simulink model "case6"  (R2024b)
settings: Solver=FixedStepAuto  StartTime=0  StopTime=1  FixedStep=1e-7  RelTol=1e-3
values from neighbouring files (symbols this model uses):
  SG_D_1_D = 0.01056    [IEEE9_case_parameters.m]    (also in case1_parameters.m; case2_parameters.m; case3_parameters.m; case4_parameters.m)
  SG_D_1_EnableSaturation = 0    [IEEE9_case_parameters.m]    (also in case1_parameters.m; case2_parameters.m; case3_parameters.m; case4_parameters.m)
  SG_D_1_f0 = 60    [IEEE9_case_parameters.m]    (also in case1_parameters.m; case2_parameters.m; case3_parameters.m; case4_parameters.m)
  SG_D_1_H = 7.5    [IEEE9_case_parameters.m]    (also in case1_parameters.m; case2_parameters.m; case3_parameters.m; case4_parameters.m)
  SG_D_1_K_A = 20    [IEEE9_case_parameters.m]    (also in case1_parameters.m; case2_parameters.m; case3_parameters.m; case4_parameters.m)
  SG_D_1_K_E = 1.000000e+1    (= 10)    [IEEE9_case_parameters.m]    (also in case1_parameters.m; case2_parameters.m; case3_parameters.m; case4_parameters.m)
  SG_D_1_K_F = 2.363    [IEEE9_case_parameters.m]    (also in case1_parameters.m; case2_parameters.m; case3_parameters.m; case4_parameters.m)
  SG_D_1_K_s = 0.5    [IEEE9_case_parameters.m]    (also in case1_parameters.m = 5; case2_parameters.m = 5; case3_parameters.m = 5; case4_parameters.m = 5)
  SG_D_1_R_a = 0.001088    [IEEE9_case_parameters.m]    (also in case1_parameters.m; case2_parameters.m; case3_parameters.m; case4_parameters.m)
  SG_D_1_S_A = 1    [IEEE9_case_parameters.m]    (also in case1_parameters.m; case2_parameters.m; case3_parameters.m; case4_parameters.m)
  SG_D_1_S_B = 0.103    [IEEE9_case_parameters.m]    (also in case1_parameters.m; case2_parameters.m; case3_parameters.m; case4_parameters.m)
  SG_D_1_S_N = 10.659857    [IEEE9_case_parameters.m]    (also in case1_parameters.m; case2_parameters.m; case3_parameters.m; case4_parameters.m)
  SG_D_1_SpeedPara = 200    [IEEE9_case_parameters.m]    (also in case1_parameters.m; case2_parameters.m; case3_parameters.m; case4_parameters.m)
  SG_D_1_T_0 = 0.720173    [IEEE9_case_parameters.m]    (also in case1_parameters.m = 0.755522; case2_parameters.m = 0.808931; case3_parameters.m = 0.869402; case4_parameters.m = 0.729316)
  SG_D_1_T_1 = 0.3    [IEEE9_case_parameters.m]    (also in case1_parameters.m; case2_parameters.m; case3_parameters.m; case4_parameters.m)
  SG_D_1_T_2 = 0.05    [IEEE9_case_parameters.m]    (also in case1_parameters.m; case2_parameters.m; case3_parameters.m; case4_parameters.m)
  SG_D_1_T_3 = 0.02    [IEEE9_case_parameters.m]    (also in case1_parameters.m; case2_parameters.m; case3_parameters.m; case4_parameters.m)
  SG_D_1_T_4 = 0.005    [IEEE9_case_parameters.m]    (also in case1_parameters.m; case2_parameters.m; case3_parameters.m; case4_parameters.m)
  SG_D_1_T_A = 0.02    [IEEE9_case_parameters.m]    (also in case1_parameters.m; case2_parameters.m; case3_parameters.m; case4_parameters.m)
  SG_D_1_T_dd = 8.000000e+0    (= 8)    [IEEE9_case_parameters.m]    (also in case1_parameters.m; case2_parameters.m; case3_parameters.m; case4_parameters.m)
  SG_D_1_T_ddd = 0.04    [IEEE9_case_parameters.m]    (also in case1_parameters.m; case2_parameters.m; case3_parameters.m; case4_parameters.m)
  SG_D_1_T_E = 0.314    [IEEE9_case_parameters.m]    (also in case1_parameters.m; case2_parameters.m; case3_parameters.m; case4_parameters.m)
  SG_D_1_T_F = 0.35    [IEEE9_case_parameters.m]    (also in case1_parameters.m; case2_parameters.m; case3_parameters.m; case4_parameters.m)
  SG_D_1_T_qd = 0.8    [IEEE9_case_parameters.m]    (also in case1_parameters.m; case2_parameters.m; case3_parameters.m; case4_parameters.m)
  SG_D_1_T_qdd = 0.02    [IEEE9_case_parameters.m]    (also in case1_parameters.m; case2_parameters.m; case3_parameters.m; case4_parameters.m)
  SG_D_1_T_speed = 0.1    [IEEE9_case_parameters.m]    (also in case1_parameters.m = 200; case2_parameters.m = 200; case3_parameters.m = 200; case4_parameters.m = 200)
  SG_D_1_T_w = 0.5    [IEEE9_case_parameters.m]    (also in case1_parameters.m; case2_parameters.m; case3_parameters.m; case4_parameters.m)
  SG_D_1_V_ref = 1.990276    [IEEE9_case_parameters.m]    (also in case1_parameters.m = 2.042296; case2_parameters.m = 2.051388; case3_parameters.m = 2.089584; case4_parameters.m = 2.01845)
  SG_D_1_w_ref = 376.991118    [IEEE9_case_parameters.m]    (also in case1_parameters.m; case2_parameters.m; case3_parameters.m; case4_parameters.m)
  SG_D_1_wb = 6.000000e+1    (= 60)    [IEEE9_case_parameters.m]    (also in case1_parameters.m; case2_parameters.m; case3_parameters.m; case4_parameters.m)
  SG_D_1_x_d = 1.9    [IEEE9_case_parameters.m]    (also in case1_parameters.m; case2_parameters.m; case3_parameters.m; case4_parameters.m)
  SG_D_1_x_dd = 0.302    [IEEE9_case_parameters.m]    (also in case1_parameters.m; case2_parameters.m; case3_parameters.m; case4_parameters.m)
  SG_D_1_x_ddd = 0.204    [IEEE9_case_parameters.m]    (also in case1_parameters.m; case2_parameters.m; case3_parameters.m; case4_parameters.m)
  SG_D_1_x_l = 0.05    [IEEE9_case_parameters.m]    (also in case1_parameters.m; case2_parameters.m; case3_parameters.m; case4_parameters.m)
  SG_D_1_x_q = 1.3    [IEEE9_case_parameters.m]    (also in case1_parameters.m; case2_parameters.m; case3_parameters.m; case4_parameters.m)
  SG_D_1_x_qd = 0.5    [IEEE9_case_parameters.m]    (also in case1_parameters.m; case2_parameters.m; case3_parameters.m; case4_parameters.m)
  SG_D_1_x_qdd = 0.3    [IEEE9_case_parameters.m]    (also in case1_parameters.m; case2_parameters.m; case3_parameters.m; case4_parameters.m)
  SG_D_2_D = 0.02    [IEEE9_case_parameters.m]    (also in case1_parameters.m; case2_parameters.m; case3_parameters.m; case4_parameters.m)
  SG_D_2_EnableSaturation = 0    [IEEE9_case_parameters.m]    (also in case1_parameters.m; case2_parameters.m; case3_parameters.m; case4_parameters.m)
  SG_D_2_f0 = 60    [IEEE9_case_parameters.m]    (also in case1_parameters.m; case2_parameters.m; case3_parameters.m; case4_parameters.m)
  SG_D_2_H = 8.000000e+0    (= 8)    [IEEE9_case_parameters.m]    (also in case1_parameters.m; case2_parameters.m; case3_parameters.m; case4_parameters.m)
  SG_D_2_K_A = 20    [IEEE9_case_parameters.m]    (also in case1_parameters.m; case2_parameters.m; case3_parameters.m; case4_parameters.m)
  SG_D_2_K_E = 1.000000e+1    (= 10)    [IEEE9_case_parameters.m]    (also in case1_parameters.m; case2_parameters.m; case3_parameters.m; case4_parameters.m)
  SG_D_2_K_F = 2.363    [IEEE9_case_parameters.m]    (also in case1_parameters.m; case2_parameters.m; case3_parameters.m; case4_parameters.m)
  SG_D_2_K_s = 0.5    [IEEE9_case_parameters.m]    (also in case1_parameters.m = 4; case2_parameters.m = 4; case3_parameters.m = 4; case4_parameters.m = 4)
  SG_D_2_R_a = 0.001088    [IEEE9_case_parameters.m]    (also in case1_parameters.m; case2_parameters.m; case3_parameters.m; case4_parameters.m)
  SG_D_2_S_A = 1    [IEEE9_case_parameters.m]    (also in case1_parameters.m; case2_parameters.m; case3_parameters.m; case4_parameters.m)
  SG_D_2_S_B = 0.103    [IEEE9_case_parameters.m]    (also in case1_parameters.m; case2_parameters.m; case3_parameters.m; case4_parameters.m)
  SG_D_2_S_N = 10.659857    [IEEE9_case_parameters.m]    (also in case1_parameters.m; case2_parameters.m; case3_parameters.m; case4_parameters.m)
  SG_D_2_SpeedPara = 200    [IEEE9_case_parameters.m]    (also in case1_parameters.m; case2_parameters.m; case3_parameters.m; case4_parameters.m)
  SG_D_2_T_0 = 1.632913    [IEEE9_case_parameters.m]    (also in case1_parameters.m = 1.632925; case2_parameters.m = 1.632915; case3_parameters.m = 1.632914; case4_parameters.m = 1.632927)
  SG_D_2_T_1 = 0.2    [IEEE9_case_parameters.m]    (also in case1_parameters.m; case2_parameters.m; case3_parameters.m; case4_parameters.m)
  SG_D_2_T_2 = 0.05    [IEEE9_case_parameters.m]    (also in case1_parameters.m; case2_parameters.m; case3_parameters.m; case4_parameters.m)
  SG_D_2_T_3 = 0.02    [IEEE9_case_parameters.m]    (also in case1_parameters.m; case2_parameters.m; case3_parameters.m; case4_parameters.m)
  SG_D_2_T_4 = 0.005    [IEEE9_case_parameters.m]    (also in case1_parameters.m; case2_parameters.m; case3_parameters.m; case4_parameters.m)
  SG_D_2_T_A = 0.02    [IEEE9_case_parameters.m]    (also in case1_parameters.m; case2_parameters.m; case3_parameters.m; case4_parameters.m)
  SG_D_2_T_dd = 7.9    [IEEE9_case_parameters.m]    (also in case1_parameters.m; case2_parameters.m; case3_parameters.m; case4_parameters.m)
  SG_D_2_T_ddd = 0.04    [IEEE9_case_parameters.m]    (also in case1_parameters.m; case2_parameters.m; case3_parameters.m; case4_parameters.m)
  SG_D_2_T_E = 0.314    [IEEE9_case_parameters.m]    (also in case1_parameters.m; case2_parameters.m; case3_parameters.m; case4_parameters.m)
  SG_D_2_T_F = 0.35    [IEEE9_case_parameters.m]    (also in case1_parameters.m; case2_parameters.m; case3_parameters.m; case4_parameters.m)
  SG_D_2_T_qd = 0.8    [IEEE9_case_parameters.m]    (also in case1_parameters.m; case2_parameters.m; case3_parameters.m; case4_parameters.m)
  SG_D_2_T_qdd = 0.015    [IEEE9_case_parameters.m]    (also in case1_parameters.m; case2_parameters.m; case3_parameters.m; case4_parameters.m)
  SG_D_2_T_speed = 0.1    [IEEE9_case_parameters.m]    (also in case1_parameters.m = 150; case2_parameters.m = 150; case3_parameters.m = 150; case4_parameters.m = 150)
  SG_D_2_T_w = 0.35    [IEEE9_case_parameters.m]    (also in case1_parameters.m; case2_parameters.m; case3_parameters.m; case4_parameters.m)
  SG_D_2_V_ref = 2.58547    [IEEE9_case_parameters.m]    (also in case1_parameters.m = 2.597896; case2_parameters.m = 2.587136; case3_parameters.m = 2.586042; case4_parameters.m = 2.599679)
  SG_D_2_w_ref = 376.991118    [IEEE9_case_parameters.m]    (also in case1_parameters.m; case2_parameters.m; case3_parameters.m; case4_parameters.m)
  SG_D_2_wb = 6.000000e+1    (= 60)    [IEEE9_case_parameters.m]    (also in case1_parameters.m; case2_parameters.m; case3_parameters.m; case4_parameters.m)
  SG_D_2_x_d = 1.8    [IEEE9_case_parameters.m]    (also in case1_parameters.m; case2_parameters.m; case3_parameters.m; case4_parameters.m)
  SG_D_2_x_dd = 0.302    [IEEE9_case_parameters.m]    (also in case1_parameters.m; case2_parameters.m; case3_parameters.m; case4_parameters.m)
  SG_D_2_x_ddd = 0.204    [IEEE9_case_parameters.m]    (also in case1_parameters.m; case2_parameters.m; case3_parameters.m; case4_parameters.m)
  SG_D_2_x_l = 0.05    [IEEE9_case_parameters.m]    (also in case1_parameters.m; case2_parameters.m; case3_parameters.m; case4_parameters.m)
  SG_D_2_x_q = 1.25    [IEEE9_case_parameters.m]    (also in case1_parameters.m; case2_parameters.m; case3_parameters.m; case4_parameters.m)
  SG_D_2_x_qd = 0.5    [IEEE9_case_parameters.m]    (also in case1_parameters.m; case2_parameters.m; case3_parameters.m; case4_parameters.m)
  SG_D_2_x_qdd = 0.3    [IEEE9_case_parameters.m]    (also in case1_parameters.m; case2_parameters.m; case3_parameters.m; case4_parameters.m)
  SG_D_3_D = 0.02    [IEEE9_case_parameters.m]    (also in case1_parameters.m; case2_parameters.m; case3_parameters.m; case4_parameters.m)
  SG_D_3_EnableSaturation = 0    [IEEE9_case_parameters.m]    (also in case1_parameters.m; case2_parameters.m; case3_parameters.m; case4_parameters.m)
  SG_D_3_f0 = 60    [IEEE9_case_parameters.m]    (also in case1_parameters.m; case2_parameters.m; case3_parameters.m; case4_parameters.m)
  SG_D_3_H = 7.7    [IEEE9_case_parameters.m]    (also in case1_parameters.m; case2_parameters.m; case3_parameters.m; case4_parameters.m)
  SG_D_3_K_A = 20    [IEEE9_case_parameters.m]    (also in case1_parameters.m; case2_parameters.m; case3_parameters.m; case4_parameters.m)
  SG_D_3_K_E = 1.000000e+1    (= 10)    [IEEE9_case_parameters.m]    (also in case1_parameters.m; case2_parameters.m; case3_parameters.m; case4_parameters.m)
  SG_D_3_K_F = 2.363    [IEEE9_case_parameters.m]    (also in case1_parameters.m; case2_parameters.m; case3_parameters.m; case4_parameters.m)
  SG_D_3_K_s = 0.2    [IEEE9_case_parameters.m]    (also in case1_parameters.m = 2; case2_parameters.m = 2; case3_parameters.m = 2; case4_parameters.m = 2)
  SG_D_3_R_a = 0.001088    [IEEE9_case_parameters.m]    (also in case1_parameters.m; case2_parameters.m; case3_parameters.m; case4_parameters.m)
  SG_D_3_S_A = 1    [IEEE9_case_parameters.m]    (also in case1_parameters.m; case2_parameters.m; case3_parameters.m; case4_parameters.m)
  SG_D_3_S_B = 0.103    [IEEE9_case_parameters.m]    (also in case1_parameters.m; case2_parameters.m; case3_parameters.m; case4_parameters.m)
  SG_D_3_S_N = 10.659857    [IEEE9_case_parameters.m]    (also in case1_parameters.m; case2_parameters.m; case3_parameters.m; case4_parameters.m)
  SG_D_3_SpeedPara = 200    [IEEE9_case_parameters.m]    (also in case1_parameters.m; case2_parameters.m; case3_parameters.m; case4_parameters.m)
  SG_D_3_T_0 = 0.850788    [IEEE9_case_parameters.m]    (also in case1_parameters.m = 0.850786; case2_parameters.m = 0.850787; case3_parameters.m; case4_parameters.m = 0.850786)
  SG_D_3_T_1 = 0.2    [IEEE9_case_parameters.m]    (also in case1_parameters.m; case2_parameters.m; case3_parameters.m; case4_parameters.m)
  SG_D_3_T_2 = 0.05    [IEEE9_case_parameters.m]    (also in case1_parameters.m; case2_parameters.m; case3_parameters.m; case4_parameters.m)
  SG_D_3_T_3 = 0.02    [IEEE9_case_parameters.m]    (also in case1_parameters.m; case2_parameters.m; case3_parameters.m; case4_parameters.m)
  SG_D_3_T_4 = 0.005    [IEEE9_case_parameters.m]    (also in case1_parameters.m; case2_parameters.m; case3_parameters.m; case4_parameters.m)
  SG_D_3_T_A = 0.02    [IEEE9_case_parameters.m]    (also in case1_parameters.m; case2_parameters.m; case3_parameters.m; case4_parameters.m)
  SG_D_3_T_dd = 8.1    [IEEE9_case_parameters.m]    (also in case1_parameters.m; case2_parameters.m; case3_parameters.m; case4_parameters.m)
  SG_D_3_T_ddd = 0.04    [IEEE9_case_parameters.m]    (also in case1_parameters.m; case2_parameters.m; case3_parameters.m; case4_parameters.m)
  SG_D_3_T_E = 0.314    [IEEE9_case_parameters.m]    (also in case1_parameters.m; case2_parameters.m; case3_parameters.m; case4_parameters.m)
  SG_D_3_T_F = 0.35    [IEEE9_case_parameters.m]    (also in case1_parameters.m; case2_parameters.m; case3_parameters.m; case4_parameters.m)
  SG_D_3_T_qd = 0.8    [IEEE9_case_parameters.m]    (also in case1_parameters.m; case2_parameters.m; case3_parameters.m; case4_parameters.m)
  SG_D_3_T_qdd = 0.015    [IEEE9_case_parameters.m]    (also in case1_parameters.m; case2_parameters.m; case3_parameters.m; case4_parameters.m)
  SG_D_3_T_speed = 0.1    [IEEE9_case_parameters.m]    (also in case1_parameters.m = 180; case2_parameters.m = 180; case3_parameters.m = 180; case4_parameters.m = 180)
  SG_D_3_T_w = 0.4    [IEEE9_case_parameters.m]    (also in case1_parameters.m; case2_parameters.m; case3_parameters.m; case4_parameters.m)
  SG_D_3_V_ref = 1.892727    [IEEE9_case_parameters.m]    (also in case1_parameters.m = 1.906439; case2_parameters.m = 1.895535; case3_parameters.m = 1.892105; case4_parameters.m = 1.906598)
  SG_D_3_w_ref = 376.991118    [IEEE9_case_parameters.m]    (also in case1_parameters.m; case2_parameters.m; case3_parameters.m; case4_parameters.m)
  SG_D_3_wb = 6.000000e+1    (= 60)    [IEEE9_case_parameters.m]    (also in case1_parameters.m; case2_parameters.m; case3_parameters.m; case4_parameters.m)
  SG_D_3_x_d = 1.85    [IEEE9_case_parameters.m]    (also in case1_parameters.m; case2_parameters.m; case3_parameters.m; case4_parameters.m)
  SG_D_3_x_dd = 0.302    [IEEE9_case_parameters.m]    (also in case1_parameters.m; case2_parameters.m; case3_parameters.m; case4_parameters.m)
  SG_D_3_x_ddd = 0.204    [IEEE9_case_parameters.m]    (also in case1_parameters.m; case2_parameters.m; case3_parameters.m; case4_parameters.m)
  SG_D_3_x_l = 0.05    [IEEE9_case_parameters.m]    (also in case1_parameters.m; case2_parameters.m; case3_parameters.m; case4_parameters.m)
  SG_D_3_x_q = 1.2    [IEEE9_case_parameters.m]    (also in case1_parameters.m; case2_parameters.m; case3_parameters.m; case4_parameters.m)
  SG_D_3_x_qd = 0.5    [IEEE9_case_parameters.m]    (also in case1_parameters.m; case2_parameters.m; case3_parameters.m; case4_parameters.m)
  SG_D_3_x_qdd = 0.3    [IEEE9_case_parameters.m]    (also in case1_parameters.m; case2_parameters.m; case3_parameters.m; case4_parameters.m)
(part 7 of 12)

== system case6/SG_D_2/T_e_SG_D_2_block ==
  note: T_e_SG_D_2 in case6
      | $-\frac{\psi _{d,\mathrm{SG},D,2}\,\left(\psi _{q,\mathrm{SG},D,2}+\frac{\psi _{\mathrm{gq},\mathrm{SG},D,2}\,\left(x_{l}-x_{\mathrm{qdd}}\right)}{x_{l}-x_{\mathrm{qd}}}+\frac{\psi _{\mathrm{kq},\mathrm{SG},D,2}\,\left(x_{\mathrm{qd}}-x_{\mathrm{qdd}}\right)}{x_{l}-x_{\mathrm{qd}}}\right)}{x_{\mathrm{qdd}}}-\frac{\psi _{q,\mathrm{SG},D,2}\,\left(\frac{\psi _{\mathrm{1d},\mathrm{SG},D,2}\,\left(x_{\mathrm{dd}}-x_{\mathrm{ddd}}\right)}{x_{\mathrm{dd}}-x_{l}}-\psi _{d,\mathrm{SG},D,2}+\frac{\psi _{\mathrm{fd},\mathrm{SG},D,2}\,\left(x_{\mathrm{ddd}}-x_{l}\right)}{x_{\mathrm{dd}}-x_{l}}\right)}{x_{\mathrm{ddd}}}$
      | Automatically generated on 2025-10-31 19:18:38 .
  State_psi_d_SG_D_2_01b1a : Inport
  State_psi_gq_SG_D_2_1bd12 : Inport  Port=2
  State_psi_kq_SG_D_2_bf31f : Inport  Port=3
  State_psi_q_SG_D_2_aa98c : Inport  Port=4
  State_psi_q_SG_D_2_0c973 : Inport  Port=5
  State_psi_1d_SG_D_2_e8fde : Inport  Port=6
  State_psi_d_SG_D_2_d0b7a : Inport  Port=7
  State_psi_fd_SG_D_2_ce60b : Inport  Port=8
  Add_2ea7c : Sum
  Add_58bf2 : Sum
  Add_62b30 : Sum
  Add_77a84 : Sum
  Add_e7f98 : Sum
  Add_ea79d : Sum
  Constant_-1_06b6f : Constant  Value=-1
  Constant_-1_114dd : Constant  Value=-1
  Constant_-1_7138b : Constant  Value=-1
  Constant_-1_a1c06 : Constant  Value=-1
  Constant_-1_a700d : Constant  Value=-1
  Constant_x_dd_42f1d : Constant  Value=x_dd
  Constant_x_dd_d85ca : Constant  Value=x_dd
  Constant_x_dd_e0bf0 : Constant  Value=x_dd
  Constant_x_ddd_1e571 : Constant  Value=x_ddd
  Constant_x_ddd_ded06 : Constant  Value=x_ddd
  Constant_x_ddd_ec3b1 : Constant  Value=x_ddd
  Constant_x_l_240e4 : Constant  Value=x_l
  Constant_x_l_3c621 : Constant  Value=x_l
  Constant_x_l_3dcae : Constant  Value=x_l
  Constant_x_l_641a0 : Constant  Value=x_l
  Constant_x_l_8f250 : Constant  Value=x_l
  Constant_x_l_c203d : Constant  Value=x_l
  Constant_x_qd_7d39f : Constant  Value=x_qd
  Constant_x_qd_7eab2 : Constant  Value=x_qd
  Constant_x_qd_8d281 : Constant  Value=x_qd
  Constant_x_qdd_04778 : Constant  Value=x_qdd
  Constant_x_qdd_c9475 : Constant  Value=x_qdd
  Constant_x_qdd_cbb36 : Constant  Value=x_qdd
  Divide_0e157 : Product  Inputs=*/
  Divide_439bb : Product  Inputs=*/
  Divide_8fe5f : Product  Inputs=*/
  Divide_9cb31 : Product  Inputs=*/
  Divide_bf510 : Product  Inputs=*/
  Divide_dccf5 : Product  Inputs=*/
  Product_0b598 : Product
  Product_45b7f : Product
  Product_57456 : Product
  Product_7b54c : Product
  Product_85705 : Product
  Product_8a2e1 : Product
  Product_978bc : Product
  Product_abe4b : Product
  Product_bbeb9 : Product
  Product_c2988 : Product
  Product_d39eb : Product
  Subtract_09de7 : Sum  Inputs=+-
  Subtract_192ee : Sum  Inputs=+-
  Subtract_23775 : Sum  Inputs=+-
  Subtract_362ee : Sum  Inputs=+-
  Subtract_5663d : Sum  Inputs=+-
  Subtract_7336a : Sum  Inputs=+-
  Subtract_ea491 : Sum  Inputs=+-
  Blockout_T_e_SG_D_2_2a19a : Outport
  wires:
  Constant_-1_7138b/1 -> Product_abe4b/1
  Divide_9cb31/1 -> Subtract_09de7/1
  Constant_-1_114dd/1 -> Product_d39eb/1
  Constant_x_l_8f250/1 -> Product_d39eb/2
  Constant_x_qd_7d39f/1 -> Subtract_362ee/1
  Product_57456/1 -> Divide_9cb31/1
  Product_d39eb/1 -> Add_58bf2/1
  Divide_8fe5f/1 -> Subtract_ea491/2
  Constant_x_qdd_c9475/1 -> Subtract_362ee/2
  Constant_x_qdd_cbb36/1 -> Divide_bf510/2
  Constant_x_ddd_ded06/1 -> Subtract_192ee/2
  Constant_x_qdd_04778/1 -> Add_58bf2/2
  Constant_x_l_240e4/1 -> Product_abe4b/2
  Constant_-1_a1c06/1 -> Product_c2988/1
  Constant_x_l_3c621/1 -> Product_c2988/2
  Constant_-1_06b6f/1 -> Product_7b54c/1
  State_psi_1d_SG_D_2_e8fde/1 -> Product_7b54c/2
  Constant_x_dd_42f1d/1 -> Subtract_192ee/1
  Divide_0e157/1 -> Subtract_09de7/2
  State_psi_gq_SG_D_2_1bd12/1 -> Product_57456/1
  Add_58bf2/1 -> Product_57456/2
  Subtract_09de7/1 -> Add_77a84/1
  Constant_x_dd_d85ca/1 -> Subtract_5663d/1
  Product_abe4b/1 -> Add_2ea7c/1
  Product_45b7f/1 -> Product_8a2e1/1
  Constant_x_qd_8d281/1 -> Add_2ea7c/2
  State_psi_kq_SG_D_2_bf31f/1 -> Product_0b598/1
  Subtract_362ee/1 -> Product_0b598/2
  Product_c2988/1 -> Add_ea79d/1
  State_psi_q_SG_D_2_0c973/1 -> Product_85705/1
  Constant_x_qd_7eab2/1 -> Add_ea79d/2
  Product_7b54c/1 -> Product_bbeb9/1
  Divide_dccf5/1 -> Add_62b30/2
  Subtract_192ee/1 -> Product_bbeb9/2
  Constant_x_l_641a0/1 -> Subtract_5663d/2
  Constant_x_ddd_1e571/1 -> Subtract_7336a/1
  Constant_x_dd_e0bf0/1 -> Subtract_23775/1
  Constant_x_l_3dcae/1 -> Subtract_7336a/2
  Add_62b30/1 -> Blockout_T_e_SG_D_2_2a19a/1
  Add_2ea7c/1 -> Divide_9cb31/2
  Product_0b598/1 -> Divide_0e157/1
  Product_8a2e1/1 -> Divide_bf510/1
  State_psi_d_SG_D_2_01b1a/1 -> Product_45b7f/2
  Add_ea79d/1 -> Divide_0e157/2
  Product_bbeb9/1 -> Divide_439bb/1
  Subtract_5663d/1 -> Divide_439bb/2
  Constant_x_l_c203d/1 -> Subtract_23775/2
  State_psi_fd_SG_D_2_ce60b/1 -> Product_978bc/1
  Constant_x_ddd_ec3b1/1 -> Divide_dccf5/2
  Product_85705/1 -> Divide_dccf5/1
  Subtract_7336a/1 -> Product_978bc/2
  Divide_439bb/1 -> Add_e7f98/1
  State_psi_d_SG_D_2_d0b7a/1 -> Add_e7f98/2
  Add_e7f98/1 -> Subtract_ea491/1
  Product_978bc/1 -> Divide_8fe5f/1
  Subtract_23775/1 -> Divide_8fe5f/2
  Constant_-1_a700d/1 -> Product_45b7f/1
  State_psi_q_SG_D_2_aa98c/1 -> Add_77a84/2
  Add_77a84/1 -> Product_8a2e1/2
  Subtract_ea491/1 -> Product_85705/2
  Divide_bf510/1 -> Add_62b30/1

== system case6/SG_D_2/d_E_fd_SG_D_2_block ==
  note: d_E_fd_SG_D_2 in case6
      | $\frac{V_{f,\mathrm{SG},D,2}-E_{\mathrm{fd},\mathrm{SG},D,2}\,K_{E}}{T_{E}}$
      | Automatically generated on 2025-10-31 19:18:17 .
  State_E_fd_SG_D_2_81070 : Inport
  State_V_f_SG_D_2_6a733 : Inport  Port=2
  Add_66f01 : Sum
  Constant_-1_dcbab : Constant  Value=-1
  Constant_K_E_07652 : Constant  Value=K_E
  Constant_T_E_566cc : Constant  Value=T_E
  Divide_9dbcd : Product  Inputs=*/
  Product_e0087 : Product
  Product_f7af1 : Product
  Blockout_d_E_fd_SG_D_2_9f684 : Outport
  wires:
  Constant_-1_dcbab/1 -> Product_f7af1/1
  State_E_fd_SG_D_2_81070/1 -> Product_f7af1/2
  Product_f7af1/1 -> Product_e0087/1
  Constant_K_E_07652/1 -> Product_e0087/2
  Product_e0087/1 -> Add_66f01/1
  Constant_T_E_566cc/1 -> Divide_9dbcd/2
  State_V_f_SG_D_2_6a733/1 -> Add_66f01/2
  Add_66f01/1 -> Divide_9dbcd/1
  Divide_9dbcd/1 -> Blockout_d_E_fd_SG_D_2_9f684/1

== system case6/SG_D_2/d_Px_1_SG_D_2_block ==
  note: d_Px_1_SG_D_2 in case6
      | $\frac{w_{\mathrm{SG},D,2}-2\,\pi \,f_{0}}{T_{w}}-\frac{\mathrm{Px}_{1,\mathrm{SG},D,2}}{T_{w}}$
      | Automatically generated on 2025-10-31 19:18:19 .
  State_Px_1_SG_D_2_84b2f : Inport
  State_w_SG_D_2_e2895 : Inport  Port=2
  Add_18d82 : Sum
  Add_71eb1 : Sum
  Constant_-1_da3fa : Constant  Value=-1
  Constant_-2.0_d7efc : Constant  Value=-2.0
  Constant_T_w_c0548 : Constant  Value=T_w
  Constant_T_w_f6b86 : Constant  Value=T_w
  Constant_f0_2a9c0 : Constant  Value=f0
  Constant_pi_ea01a : Constant  Value=pi
  Divide_ba524 : Product  Inputs=*/
  Divide_bd779 : Product  Inputs=*/
  Product_269cd : Product
  Product_9781d : Product
  Product_f6073 : Product
  Blockout_d_Px_1_SG_D_2_cd7c4 : Outport
  wires:
  Constant_-2.0_d7efc/1 -> Product_9781d/1
  State_w_SG_D_2_e2895/1 -> Add_71eb1/2
  Constant_pi_ea01a/1 -> Product_9781d/2
  Product_9781d/1 -> Product_f6073/1
  Constant_f0_2a9c0/1 -> Product_f6073/2
  Constant_-1_da3fa/1 -> Product_269cd/1
  State_Px_1_SG_D_2_84b2f/1 -> Product_269cd/2
  Product_f6073/1 -> Add_71eb1/1
  Product_269cd/1 -> Divide_ba524/1
  Constant_T_w_c0548/1 -> Divide_ba524/2
  Add_71eb1/1 -> Divide_bd779/1
  Constant_T_w_f6b86/1 -> Divide_bd779/2
  Divide_ba524/1 -> Add_18d82/1
  Divide_bd779/1 -> Add_18d82/2
  Add_18d82/1 -> Blockout_d_Px_1_SG_D_2_cd7c4/1

== system case6/SG_D_2/d_Px_2_SG_D_2_block ==
  note: d_Px_2_SG_D_2 in case6
      | $\frac{\mathrm{Px}_{1,\mathrm{SG},D,2}-T_{2}\,\left(\frac{\mathrm{Px}_{1,\mathrm{SG},D,2}}{T_{w}}-\frac{w_{\mathrm{SG},D,2}-2\,\pi \,f_{0}}{T_{w}}\right)}{T_{1}}-\frac{\mathrm{Px}_{2,\mathrm{SG},D,2}}{T_{1}}$
      | Automatically generated on 2025-10-31 19:18:21 .
  State_Px_2_SG_D_2_b5883 : Inport
  State_Px_1_SG_D_2_b4148 : Inport  Port=2
  State_Px_1_SG_D_2_e0226 : Inport  Port=3
  State_w_SG_D_2_c3292 : Inport  Port=4
  Add_acb0b : Sum
  Add_c54a1 : Sum
  Add_ec9e4 : Sum
  Add_ef894 : Sum
  Constant_-1_09813 : Constant  Value=-1
  Constant_-1_b0410 : Constant  Value=-1
  Constant_-2.0_dd1ee : Constant  Value=-2.0
  Constant_T_1_4098a : Constant  Value=T_1
  Constant_T_1_e9764 : Constant  Value=T_1
  Constant_T_2_da471 : Constant  Value=T_2
  Constant_T_w_adc65 : Constant  Value=T_w
  Constant_T_w_dc48d : Constant  Value=T_w
  Constant_f0_eaacf : Constant  Value=f0
  Constant_pi_2505b : Constant  Value=pi
  Divide_09629 : Product  Inputs=*/
  Divide_8e036 : Product  Inputs=*/
  Divide_94c1d : Product  Inputs=*/
  Divide_fbf7a : Product  Inputs=*/
  Product_22ec6 : Product
  Product_ae225 : Product
  Product_de082 : Product
  Product_e764e : Product
  Product_f78aa : Product
  Blockout_d_Px_2_SG_D_2_75597 : Outport
  wires:
  Constant_-1_09813/1 -> Product_f78aa/1
  Constant_-2.0_dd1ee/1 -> Product_ae225/1
  Product_22ec6/1 -> Add_ef894/2
  State_w_SG_D_2_c3292/1 -> Add_ec9e4/2
  Constant_pi_2505b/1 -> Product_ae225/2
  Product_ae225/1 -> Product_e764e/1
  State_Px_1_SG_D_2_e0226/1 -> Product_de082/2
  Constant_f0_eaacf/1 -> Product_e764e/2
  State_Px_2_SG_D_2_b5883/1 -> Product_f78aa/2
  Constant_-1_b0410/1 -> Product_de082/1
  Product_e764e/1 -> Add_ec9e4/1
  Product_de082/1 -> Divide_94c1d/1
  Constant_T_w_dc48d/1 -> Divide_94c1d/2
  Add_ec9e4/1 -> Divide_8e036/1
  Constant_T_w_adc65/1 -> Divide_8e036/2
  Divide_94c1d/1 -> Add_acb0b/1
  Divide_8e036/1 -> Add_acb0b/2
  Constant_T_2_da471/1 -> Product_22ec6/1
  Add_acb0b/1 -> Product_22ec6/2
  State_Px_1_SG_D_2_b4148/1 -> Add_ef894/1
  Product_f78aa/1 -> Divide_fbf7a/1
  Constant_T_1_4098a/1 -> Divide_fbf7a/2
  Add_ef894/1 -> Divide_09629/1
  Constant_T_1_e9764/1 -> Divide_09629/2
  Divide_fbf7a/1 -> Add_c54a1/1
  Divide_09629/1 -> Add_c54a1/2
  Add_c54a1/1 -> Blockout_d_Px_2_SG_D_2_75597/1

== system case6/SG_D_2/d_Px_3_SG_D_2_block ==
  note: d_Px_3_SG_D_2 in case6
      | $\frac{\mathrm{Px}_{2,\mathrm{SG},D,2}+T_{4}\,\left(\frac{\mathrm{Px}_{1,\mathrm{SG},D,2}-T_{2}\,\left(\frac{\mathrm{Px}_{1,\mathrm{SG},D,2}}{T_{w}}-\frac{w_{\mathrm{SG},D,2}-2\,\pi \,f_{0}}{T_{w}}\right)}{T_{1}}-\frac{\mathrm{Px}_{2,\mathrm{SG},D,2}}{T_{1}}\right)}{T_{3}}-\frac{\mathrm{Px}_{3,\mathrm{SG},D,2}}{T_{3}}$
      | Automatically generated on 2025-10-31 19:18:23 .
  State_Px_3_SG_D_2_5e818 : Inport
  State_Px_2_SG_D_2_d06b1 : Inport  Port=2
  State_Px_2_SG_D_2_72320 : Inport  Port=3
  State_Px_1_SG_D_2_bdfda : Inport  Port=4
  State_Px_1_SG_D_2_c353d : Inport  Port=5
  State_w_SG_D_2_e2d04 : Inport  Port=6
  Add_2957c : Sum
  Add_d3b52 : Sum
  Add_e80c4 : Sum
  Add_ed1e1 : Sum
  Add_f1cd5 : Sum
  Add_fdd0c : Sum
  Constant_-1_18dbe : Constant  Value=-1
  Constant_-1_2f44a : Constant  Value=-1
  Constant_-1_e3252 : Constant  Value=-1
  Constant_-2.0_81b8f : Constant  Value=-2.0
  Constant_T_1_0689f : Constant  Value=T_1
  Constant_T_1_40c17 : Constant  Value=T_1
  Constant_T_2_3aed3 : Constant  Value=T_2
  Constant_T_3_3da07 : Constant  Value=T_3
  Constant_T_3_cac9f : Constant  Value=T_3
  Constant_T_4_0831b : Constant  Value=T_4
  Constant_T_w_54d38 : Constant  Value=T_w
  Constant_T_w_ffad6 : Constant  Value=T_w
  Constant_f0_e635b : Constant  Value=f0
  Constant_pi_e5711 : Constant  Value=pi
  Divide_17eed : Product  Inputs=*/
  Divide_60777 : Product  Inputs=*/
  Divide_70df4 : Product  Inputs=*/
  Divide_c4777 : Product  Inputs=*/
  Divide_f98fb : Product  Inputs=*/
  Divide_fb71f : Product  Inputs=*/
  Product_2e138 : Product
  Product_30222 : Product
  Product_549d0 : Product
  Product_577a3 : Product
  Product_6a335 : Product
  Product_dfaed : Product
  Product_f7a9c : Product
  Blockout_d_Px_3_SG_D_2_4fae6 : Outport
  wires:
  Constant_-2.0_81b8f/1 -> Product_577a3/1
  State_w_SG_D_2_e2d04/1 -> Add_ed1e1/2
  Add_e80c4/1 -> Divide_f98fb/1
  Constant_pi_e5711/1 -> Product_577a3/2
  Constant_-1_2f44a/1 -> Product_30222/1
  Product_577a3/1 -> Product_2e138/1
  State_Px_2_SG_D_2_72320/1 -> Product_30222/2
  State_Px_1_SG_D_2_c353d/1 -> Product_549d0/2
  Divide_f98fb/1 -> Add_d3b52/2
  Constant_f0_e635b/1 -> Product_2e138/2
  Constant_-1_e3252/1 -> Product_549d0/1
  Product_2e138/1 -> Add_ed1e1/1
  Product_549d0/1 -> Divide_60777/1
  Constant_T_w_54d38/1 -> Divide_60777/2
  Divide_fb71f/1 -> Add_d3b52/1
  Add_ed1e1/1 -> Divide_70df4/1
  Product_f7a9c/1 -> Add_fdd0c/2
  Constant_T_w_ffad6/1 -> Divide_70df4/2
  Divide_60777/1 -> Add_f1cd5/1
  State_Px_1_SG_D_2_bdfda/1 -> Add_fdd0c/1
  Divide_70df4/1 -> Add_f1cd5/2
  Constant_-1_18dbe/1 -> Product_6a335/1
  Constant_T_2_3aed3/1 -> Product_f7a9c/1
  Add_f1cd5/1 -> Product_f7a9c/2
  Product_30222/1 -> Divide_c4777/1
  Constant_T_1_0689f/1 -> Divide_c4777/2
  Add_fdd0c/1 -> Divide_17eed/1
  Constant_T_1_40c17/1 -> Divide_17eed/2
  Divide_c4777/1 -> Add_2957c/1
  Divide_17eed/1 -> Add_2957c/2
  Constant_T_4_0831b/1 -> Product_dfaed/1
  Add_2957c/1 -> Product_dfaed/2
  State_Px_3_SG_D_2_5e818/1 -> Product_6a335/2
  State_Px_2_SG_D_2_d06b1/1 -> Add_e80c4/1
  Product_dfaed/1 -> Add_e80c4/2
  Product_6a335/1 -> Divide_fb71f/1
  Constant_T_3_cac9f/1 -> Divide_fb71f/2
  Constant_T_3_3da07/1 -> Divide_f98fb/2
  Add_d3b52/1 -> Blockout_d_Px_3_SG_D_2_4fae6/1

== system case6/SG_D_2/d_R_f_SG_D_2_block ==
  note: d_R_f_SG_D_2 in case6
      | $-\frac{R_{f,\mathrm{SG},D,2}-\frac{E_{\mathrm{fd},\mathrm{SG},D,2}\,K_{F}}{T_{F}}}{T_{F}}$
      | Automatically generated on 2025-10-31 19:18:16 .
  State_E_fd_SG_D_2_5e385 : Inport
  State_R_f_SG_D_2_02ca4 : Inport  Port=2
  Constant_K_F_a1dcc : Constant  Value=K_F
  Constant_T_F_2ae9d : Constant  Value=T_F
  Constant_T_F_533cd : Constant  Value=T_F
  Divide_13ef8 : Product  Inputs=*/
  Divide_f44b1 : Product  Inputs=*/
  Product_38810 : Product
  Subtract_39a00 : Sum  Inputs=+-
  Blockout_d_R_f_SG_D_2_cc0fa : Outport
  wires:
  Constant_T_F_533cd/1 -> Divide_13ef8/2
  State_E_fd_SG_D_2_5e385/1 -> Product_38810/1
  Constant_K_F_a1dcc/1 -> Product_38810/2
  State_R_f_SG_D_2_02ca4/1 -> Subtract_39a00/2
  Product_38810/1 -> Divide_13ef8/1
  Divide_13ef8/1 -> Subtract_39a00/1
  Constant_T_F_2ae9d/1 -> Divide_f44b1/2
  Subtract_39a00/1 -> Divide_f44b1/1
  Divide_f44b1/1 -> Blockout_d_R_f_SG_D_2_cc0fa/1

== system case6/SG_D_2/d_T_m_SG_D_2_block ==
  note: d_T_m_SG_D_2 in case6
      | $-\frac{T_{m,\mathrm{SG},D,2}-T_{0}+\frac{\mathrm{SpeedPara}\,\left(w_{\mathrm{SG},D,2}-w_{\mathrm{ref}}\right)}{2\,f_{0}\,\pi }}{T_{\mathrm{speed}}}$
      | Automatically generated on 2025-10-31 19:18:05 .
  State_w_SG_D_2_d1516 : Inport
  State_T_m_SG_D_2_36b08 : Inport  Port=2
  Add_0784f : Sum
  Add_6913c : Sum
  Constant_-1_1a06d : Constant  Value=-1
  Constant_2.0_5a98b : Constant  Value=2.0
  Constant_SpeedPara_c4dfb : Constant  Value=SpeedPara
  Constant_T_0_6e352 : Constant  Value=T_0
  Constant_T_speed_98489 : Constant  Value=T_speed
  Constant_f0_d2b83 : Constant  Value=f0
  Constant_pi_c158b : Constant  Value=pi
  Constant_w_ref_cd502 : Constant  Value=w_ref
  Divide_2fe7c : Product  Inputs=*/
  Divide_b72ab : Product  Inputs=*/
  Product_0bae0 : Product
  Product_9c6b5 : Product
  Product_b6a36 : Product
  Product_fdb7b : Product
  Subtract_7f6d6 : Sum  Inputs=+-
  Blockout_d_T_m_SG_D_2_8c4dc : Outport
  wires:
  Constant_pi_c158b/1 -> Product_9c6b5/2
  Constant_-1_1a06d/1 -> Product_0bae0/1
  Constant_w_ref_cd502/1 -> Add_0784f/2
  State_w_SG_D_2_d1516/1 -> Product_0bae0/2
  Product_0bae0/1 -> Add_0784f/1
  Add_6913c/1 -> Subtract_7f6d6/1
  Add_0784f/1 -> Product_fdb7b/2
  Constant_2.0_5a98b/1 -> Product_9c6b5/1
  Constant_SpeedPara_c4dfb/1 -> Product_fdb7b/1
  Product_9c6b5/1 -> Product_b6a36/1
  Constant_f0_d2b83/1 -> Product_b6a36/2
  Product_fdb7b/1 -> Divide_2fe7c/1
  Product_b6a36/1 -> Divide_2fe7c/2
  Divide_2fe7c/1 -> Add_6913c/1
  Constant_T_0_6e352/1 -> Add_6913c/2
  State_T_m_SG_D_2_36b08/1 -> Subtract_7f6d6/2
  Subtract_7f6d6/1 -> Divide_b72ab/1
  Constant_T_speed_98489/1 -> Divide_b72ab/2
  Divide_b72ab/1 -> Blockout_d_T_m_SG_D_2_8c4dc/1

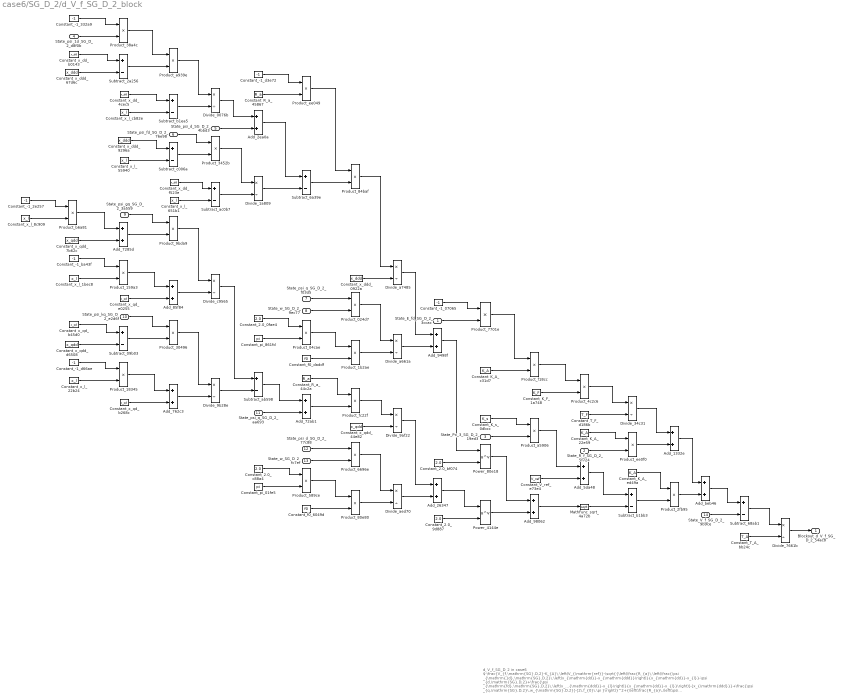
== system case6/SG_D_2/d_V_f_SG_D_2_block ==
  note: d_V_f_SG_D_2 in case6
      | $-\frac{V_{f,\mathrm{SG},D,2}-K_{A}\,\left(V_{\mathrm{ref}}-\sqrt{{\left(\frac{R_{a}\,\left(\frac{\psi _{\mathrm{1d},\mathrm{SG},D,2}\,\left(x_{\mathrm{dd}}-x_{\mathrm{ddd}}\right)}{x_{\mathrm{dd}}-x_{l}}-\psi _{d,\mathrm{SG},D,2}+\frac{\psi _{\mathrm{fd},\mathrm{SG},D,2}\,\left(x_{\mathrm{ddd}}-x_{l}\right)}{x_{\mathrm{dd}}-x_{l}}\right)}{x_{\mathrm{ddd}}}+\frac{\psi _{q,\mathrm{SG},D,2}\,w_{\mathrm{SG},D,2}}{2\,f_{0}\,\pi }\right)}^2+{\left(\frac{R_{a}\,\left(\psi _{q,\mathrm{SG},D,2}+\frac{\psi _{\mathrm{gq},\mathrm{SG},D,2}\,\left(x_{l}-x_{\mathrm{qdd}}\right)}{x_{l}-x_{\mathrm{qd}}}+\frac{\psi _{\mathrm{kq},\mathrm{SG},D,2}\,\left(x_{\mathrm{qd}}-x_{\mathrm{qdd}}\right)}{x_{l}-x_{\mathrm{qd}}}\right)}{x_{\mathrm{qdd}}}+\frac{\psi _{d,\mathrm{SG},D,2}\,w_{\mathrm{SG},D,2}}{2\,f_{0}\,\pi }\right)}^2}+K_{s}\,\mathrm{Px}_{3,\mathrm{SG},D,2}\right)-K_{A}\,R_{f,\mathrm{SG},D,2}+\frac{E_{\mathrm{fd},\mathrm{SG},D,2}\,K_{A}\,K_{F}}{T_{F}}}{T_{A}}$
      | Automatically generated on 2025-10-31 19:18:14 .
  State_E_fd_SG_D_2_3ccac : Inport
  State_R_f_SG_D_2_5f724 : Inport  Port=2
  State_Px_3_SG_D_2_19ed3 : Inport  Port=3
  State_psi_1d_SG_D_2_d8f0b : Inport  Port=4
  State_psi_d_SG_D_2_4bbd3 : Inport  Port=5
  State_psi_fd_SG_D_2_76e98 : Inport  Port=6
  State_psi_q_SG_D_2_f03d5 : Inport  Port=7
  State_w_SG_D_2_9ec77 : Inport  Port=8
  State_psi_gq_SG_D_2_3a559 : Inport  Port=9
  State_psi_kq_SG_D_2_e2d6f : Inport  Port=10
  State_psi_q_SG_D_2_aa693 : Inport  Port=11
  State_psi_d_SG_D_2_77c88 : Inport  Port=12
  State_w_SG_D_2_fc7ef : Inport  Port=13
  State_V_f_SG_D_2_9b9ce : Inport  Port=14
  Add_1332e : Sum
  Add_26347 : Sum
  Add_2ea0a : Sum
  Add_5da48 : Sum
  Add_7285d : Sum
  Add_72ab1 : Sum
  Add_762c3 : Sum
  Add_85f84 : Sum
  Add_9498f : Sum
  Add_98062 : Sum
  Add_beb46 : Sum
  Constant_-1_07065 : Constant  Value=-1
  Constant_-1_2e257 : Constant  Value=-1
  Constant_-1_332a9 : Constant  Value=-1
  Constant_-1_ba43f : Constant  Value=-1
  Constant_-1_d3e72 : Constant  Value=-1
  Constant_-1_d66ae : Constant  Value=-1
  Constant_2.0_0fae4 : Constant  Value=2.0
  Constant_2.0_9d887 : Constant  Value=2.0
  Constant_2.0_bf074 : Constant  Value=2.0
  Constant_2.0_c88a4 : Constant  Value=2.0
  Constant_K_A_22e59 : Constant  Value=K_A
  Constant_K_A_c31d7 : Constant  Value=K_A
  Constant_K_A_ed49a : Constant  Value=K_A
  Constant_K_F_1a748 : Constant  Value=K_F
  Constant_K_s_0dbcc : Constant  Value=K_s
  Constant_R_a_44c2a : Constant  Value=R_a
  Constant_R_a_45867 : Constant  Value=R_a
  Constant_T_A_bb24c : Constant  Value=T_A
  Constant_T_F_d186b : Constant  Value=T_F
  Constant_V_ref_e73e4 : Constant  Value=V_ref
  Constant_f0_6049d : Constant  Value=f0
  Constant_f0_daddf : Constant  Value=f0
  Constant_pi_01fe5 : Constant  Value=pi
  Constant_pi_861fd : Constant  Value=pi
  Constant_x_dd_4cec5 : Constant  Value=x_dd
  Constant_x_dd_b0143 : Constant  Value=x_dd
  Constant_x_dd_f523e : Constant  Value=x_dd
  Constant_x_ddd_0922a : Constant  Value=x_ddd
  Constant_x_ddd_67d6c : Constant  Value=x_ddd
  Constant_x_ddd_9296a : Constant  Value=x_ddd
  Constant_x_l_1bec8 : Constant  Value=x_l
  Constant_x_l_22b24 : Constant  Value=x_l
  Constant_x_l_55940 : Constant  Value=x_l
  Constant_x_l_651b1 : Constant  Value=x_l
  Constant_x_l_8c909 : Constant  Value=x_l
  Constant_x_l_cb82e : Constant  Value=x_l
  Constant_x_qd_b268c : Constant  Value=x_qd
  Constant_x_qd_b45d0 : Constant  Value=x_qd
  Constant_x_qd_e0255 : Constant  Value=x_qd
  Constant_x_qdd_44e82 : Constant  Value=x_qdd
  Constant_x_qdd_7b62c : Constant  Value=x_qdd
  Constant_x_qdd_d6508 : Constant  Value=x_qdd
  Divide_0076b : Product  Inputs=*/
  Divide_1a809 : Product  Inputs=*/
  Divide_34c31 : Product  Inputs=*/
  Divide_7661b : Product  Inputs=*/
  Divide_9af22 : Product  Inputs=*/
  Divide_9b28e : Product  Inputs=*/
  Divide_a661a : Product  Inputs=*/
  Divide_a7485 : Product  Inputs=*/
  Divide_aed70 : Product  Inputs=*/
  Divide_c9565 : Product  Inputs=*/
  MathFunc_sqrt_4a72b : Sqrt
  Power_4144e : Math  Operator=pow
  Power_80e18 : Math  Operator=pow
  Product_024d7 : Product
  Product_04cae : Product
  Product_159a3 : Product
  Product_18345 : Product
  Product_1b2ae : Product
  Product_2fb95 : Product
  Product_30496 : Product
  Product_3452b : Product
  Product_38a4c : Product
  Product_4c2c6 : Product
  Product_589ce : Product
  Product_6696e : Product
  Product_7701e : Product
  Product_80e80 : Product
  Product_84baf : Product
  Product_9bda9 : Product
  Product_a5906 : Product
  Product_a939e : Product
  Product_b6a81 : Product
  Product_ee049 : Product
  Product_ee0f0 : Product
  Product_f18cc : Product
  Product_fc22f : Product
  Subtract_09b03 : Sum  Inputs=+-
  Subtract_2a256 : Sum  Inputs=+-
  Subtract_68ab1 : Sum  Inputs=+-
  Subtract_6a39e : Sum  Inputs=+-
  Subtract_ab598 : Sum  Inputs=+-
  Subtract_ac0b7 : Sum  Inputs=+-
  Subtract_b1bb3 : Sum  Inputs=+-
  Subtract_b1ea5 : Sum  Inputs=+-
  Subtract_c006a : Sum  Inputs=+-
  Blockout_d_V_f_SG_D_2_54ac8 : Outport
  wires:
  Constant_-1_332a9/1 -> Product_38a4c/1
  Constant_2.0_0fae4/1 -> Product_04cae/1
  Constant_-1_2e257/1 -> Product_b6a81/1
  Product_04cae/1 -> Product_1b2ae/1
  Product_b6a81/1 -> Add_7285d/1
  Constant_x_l_22b24/1 -> Product_18345/2
  Constant_x_l_8c909/1 -> Product_b6a81/2
  State_psi_1d_SG_D_2_d8f0b/1 -> Product_38a4c/2
  Constant_x_l_651b1/1 -> Subtract_ac0b7/2
  Constant_x_dd_b0143/1 -> Subtract_2a256/1
  Product_fc22f/1 -> Divide_9af22/1
  Constant_x_ddd_67d6c/1 -> Subtract_2a256/2
  Constant_x_qd_b268c/1 -> Add_762c3/2
  Add_7285d/1 -> Product_9bda9/2
  Constant_x_qdd_7b62c/1 -> Add_7285d/2
  Constant_-1_ba43f/1 -> Product_159a3/1
  Constant_x_dd_f523e/1 -> Subtract_ac0b7/1
  Subtract_ab598/1 -> Add_72ab1/1
  Power_80e18/1 -> Add_98062/1
  Constant_x_l_1bec8/1 -> Product_159a3/2
  Constant_2.0_c88a4/1 -> Product_589ce/1
  Constant_x_qd_b45d0/1 -> Subtract_09b03/1
  Constant_pi_01fe5/1 -> Product_589ce/2
  Subtract_6a39e/1 -> Product_84baf/2
  Constant_x_qdd_d6508/1 -> Subtract_09b03/2
  State_psi_fd_SG_D_2_76e98/1 -> Product_3452b/1
  Constant_-1_d66ae/1 -> Product_18345/1
  Product_38a4c/1 -> Product_a939e/1
  State_w_SG_D_2_fc7ef/1 -> Product_6696e/2
  Subtract_2a256/1 -> Product_a939e/2
  Constant_x_dd_4cec5/1 -> Subtract_b1ea5/1
  State_psi_q_SG_D_2_aa693/1 -> Add_72ab1/2
  State_w_SG_D_2_9ec77/1 -> Product_024d7/2
  Subtract_c006a/1 -> Product_3452b/2
  Constant_x_l_cb82e/1 -> Subtract_b1ea5/2
  Add_1332e/1 -> Add_beb46/1
  Constant_x_ddd_9296a/1 -> Subtract_c006a/1
  Constant_x_l_55940/1 -> Subtract_c006a/2
  State_psi_gq_SG_D_2_3a559/1 -> Product_9bda9/1
  Product_159a3/1 -> Add_85f84/1
  Subtract_ac0b7/1 -> Divide_1a809/2
  Constant_x_qd_e0255/1 -> Add_85f84/2
  Product_024d7/1 -> Divide_a661a/1
  State_psi_kq_SG_D_2_e2d6f/1 -> Product_30496/1
  Subtract_09b03/1 -> Product_30496/2
  Product_3452b/1 -> Divide_1a809/1
  State_V_f_SG_D_2_9b9ce/1 -> Subtract_68ab1/2
  Product_18345/1 -> Add_762c3/1
  Product_a939e/1 -> Divide_0076b/1
  Divide_c9565/1 -> Subtract_ab598/1
  Subtract_b1ea5/1 -> Divide_0076b/2
  Product_9bda9/1 -> Divide_c9565/1
  Add_85f84/1 -> Divide_c9565/2
  Product_30496/1 -> Divide_9b28e/1
  Divide_1a809/1 -> Subtract_6a39e/2
  Constant_f0_daddf/1 -> Product_1b2ae/2
  Add_762c3/1 -> Divide_9b28e/2
  Divide_0076b/1 -> Add_2ea0a/1
  State_psi_d_SG_D_2_4bbd3/1 -> Add_2ea0a/2
  Divide_9b28e/1 -> Subtract_ab598/2
  Constant_-1_d3e72/1 -> Product_ee049/1
  Constant_R_a_45867/1 -> Product_ee049/2
  Constant_f0_6049d/1 -> Product_80e80/2
  Add_2ea0a/1 -> Subtract_6a39e/1
  Product_ee049/1 -> Product_84baf/1
  Constant_pi_861fd/1 -> Product_04cae/2
  State_psi_q_SG_D_2_f03d5/1 -> Product_024d7/1
  Constant_R_a_44c2a/1 -> Product_fc22f/1
  State_E_fd_SG_D_2_3ccac/1 -> Product_7701e/2
  Add_72ab1/1 -> Product_fc22f/2
  State_psi_d_SG_D_2_77c88/1 -> Product_6696e/1
  Product_589ce/1 -> Product_80e80/1
  Product_84baf/1 -> Divide_a7485/1
  Constant_x_ddd_0922a/1 -> Divide_a7485/2
  Product_1b2ae/1 -> Divide_a661a/2
  Constant_x_qdd_44e82/1 -> Divide_9af22/2
  Product_6696e/1 -> Divide_aed70/1
  Product_80e80/1 -> Divide_aed70/2
  Divide_a7485/1 -> Add_9498f/1
  Divide_a661a/1 -> Add_9498f/2
  Divide_9af22/1 -> Add_26347/1
  Divide_aed70/1 -> Add_26347/2
  Constant_-1_07065/1 -> Product_7701e/1
  Add_9498f/1 -> Power_80e18/1
  Constant_2.0_bf074/1 -> Power_80e18/2
  Add_26347/1 -> Power_4144e/1
  Constant_2.0_9d887/1 -> Power_4144e/2
  Product_7701e/1 -> Product_f18cc/1
  Constant_K_A_c31d7/1 -> Product_f18cc/2
  Constant_K_s_0dbcc/1 -> Product_a5906/1
  State_Px_3_SG_D_2_19ed3/1 -> Product_a5906/2
  Power_4144e/1 -> Add_98062/2
  Product_f18cc/1 -> Product_4c2c6/1
  Constant_K_F_1a748/1 -> Product_4c2c6/2
  Product_a5906/1 -> Add_5da48/1
  Constant_V_ref_e73e4/1 -> Add_5da48/2
  Add_98062/1 -> MathFunc_sqrt_4a72b/1
  Product_4c2c6/1 -> Divide_34c31/1
  Constant_T_F_d186b/1 -> Divide_34c31/2
  Constant_K_A_22e59/1 -> Product_ee0f0/1
  State_R_f_SG_D_2_5f724/1 -> Product_ee0f0/2
  Add_5da48/1 -> Subtract_b1bb3/1
  MathFunc_sqrt_4a72b/1 -> Subtract_b1bb3/2
  Divide_34c31/1 -> Add_1332e/1
  Product_ee0f0/1 -> Add_1332e/2
  Constant_K_A_ed49a/1 -> Product_2fb95/1
  Subtract_b1bb3/1 -> Product_2fb95/2
  Product_2fb95/1 -> Add_beb46/2
  Add_beb46/1 -> Subtract_68ab1/1
  Subtract_68ab1/1 -> Divide_7661b/1
  Constant_T_A_bb24c/1 -> Divide_7661b/2
  Divide_7661b/1 -> Blockout_d_V_f_SG_D_2_54ac8/1

== system case6/SG_D_2/d_psi_1d_SG_D_2_block ==
  note: d_psi_1d_SG_D_2 in case6
      | $-\frac{\psi _{\mathrm{1d},\mathrm{SG},D,2}-\psi _{\mathrm{fd},\mathrm{SG},D,2}+\frac{\left(x_{\mathrm{dd}}-x_{l}\right)\,\left(\frac{\psi _{\mathrm{1d},\mathrm{SG},D,2}\,\left(x_{\mathrm{dd}}-x_{\mathrm{ddd}}\right)}{x_{\mathrm{dd}}-x_{l}}-\psi _{d,\mathrm{SG},D,2}+\frac{\psi _{\mathrm{fd},\mathrm{SG},D,2}\,\left(x_{\mathrm{ddd}}-x_{l}\right)}{x_{\mathrm{dd}}-x_{l}}\right)}{x_{\mathrm{ddd}}}}{T_{\mathrm{ddd}}}$
      | Automatically generated on 2025-10-31 19:17:45 .
  State_psi_1d_SG_D_2_5b9a9 : Inport
  State_psi_fd_SG_D_2_5c5ab : Inport  Port=2
  State_psi_1d_SG_D_2_2957b : Inport  Port=3
  State_psi_d_SG_D_2_2211c : Inport  Port=4
  State_psi_fd_SG_D_2_68d1a : Inport  Port=5
  Add_3ea78 : Sum
  Add_50738 : Sum
  Add_929bd : Sum
  Constant_-1_771c4 : Constant  Value=-1
  Constant_-1_fb906 : Constant  Value=-1
  Constant_T_ddd_c4547 : Constant  Value=T_ddd
  Constant_x_dd_02b01 : Constant  Value=x_dd
  Constant_x_dd_67da2 : Constant  Value=x_dd
  Constant_x_dd_be23a : Constant  Value=x_dd
  Constant_x_dd_d2b43 : Constant  Value=x_dd
  Constant_x_ddd_60ac6 : Constant  Value=x_ddd
  Constant_x_ddd_b41cb : Constant  Value=x_ddd
  Constant_x_ddd_f61c4 : Constant  Value=x_ddd
  Constant_x_l_3560f : Constant  Value=x_l
  Constant_x_l_5a297 : Constant  Value=x_l
  Constant_x_l_e08d0 : Constant  Value=x_l
  Constant_x_l_f82b2 : Constant  Value=x_l
  Divide_0202b : Product  Inputs=*/
  Divide_12e41 : Product  Inputs=*/
  Divide_339a9 : Product  Inputs=*/
  Divide_c3513 : Product  Inputs=*/
  Product_0684f : Product
  Product_6a5af : Product
  Product_add5f : Product
  Product_de88d : Product
  Product_ef236 : Product
  Subtract_3007f : Sum  Inputs=+-
  Subtract_31875 : Sum  Inputs=+-
  Subtract_4deb0 : Sum  Inputs=+-
  Subtract_9cec7 : Sum  Inputs=+-
  Subtract_b2f58 : Sum  Inputs=+-
  Subtract_f7f6a : Sum  Inputs=+-
  Blockout_d_psi_1d_SG_D_2_a3cd5 : Outport
  wires:
  Subtract_3007f/1 -> Product_add5f/2
  Constant_x_l_5a297/1 -> Subtract_b2f58/2
  Divide_0202b/1 -> Add_3ea78/2
  Subtract_4deb0/1 -> Product_6a5af/2
  Constant_-1_771c4/1 -> Product_de88d/1
  Constant_x_dd_d2b43/1 -> Subtract_31875/1
  Divide_339a9/1 -> Blockout_d_psi_1d_SG_D_2_a3cd5/1
  State_psi_fd_SG_D_2_5c5ab/1 -> Add_50738/2
  State_psi_1d_SG_D_2_2957b/1 -> Product_de88d/2
  Divide_c3513/1 -> Subtract_4deb0/2
  Constant_x_ddd_b41cb/1 -> Subtract_31875/2
  State_psi_1d_SG_D_2_5b9a9/1 -> Product_0684f/2
  Product_de88d/1 -> Product_ef236/1
  Subtract_31875/1 -> Product_ef236/2
  Constant_x_dd_02b01/1 -> Subtract_b2f58/1
  Constant_x_ddd_f61c4/1 -> Subtract_3007f/1
  Constant_x_l_3560f/1 -> Subtract_3007f/2
  Product_ef236/1 -> Divide_12e41/1
  Subtract_b2f58/1 -> Divide_12e41/2
  State_psi_fd_SG_D_2_68d1a/1 -> Product_add5f/1
  Constant_x_dd_be23a/1 -> Subtract_9cec7/1
  Constant_x_l_f82b2/1 -> Subtract_f7f6a/2
  Constant_x_l_e08d0/1 -> Subtract_9cec7/2
  Constant_x_ddd_60ac6/1 -> Divide_0202b/2
  Divide_12e41/1 -> Add_929bd/1
  State_psi_d_SG_D_2_2211c/1 -> Add_929bd/2
  Product_add5f/1 -> Divide_c3513/1
  Subtract_9cec7/1 -> Divide_c3513/2
  Constant_x_dd_67da2/1 -> Subtract_f7f6a/1
  Add_929bd/1 -> Subtract_4deb0/1
  Constant_-1_fb906/1 -> Product_0684f/1
  Subtract_f7f6a/1 -> Product_6a5af/1
  Product_0684f/1 -> Add_50738/1
  Product_6a5af/1 -> Divide_0202b/1
  Add_50738/1 -> Add_3ea78/1
  Add_3ea78/1 -> Divide_339a9/1
  Constant_T_ddd_c4547/1 -> Divide_339a9/2
